simulink model "realtimeE4"  (R2024b)
settings: Solver=VariableStepAuto  StartTime=0.0  StopTime=10.0  RelTol=1e-3
values from neighbouring files (symbols this model uses):
  C = Tc/(Tc+Ts)    [Observer_and_complementary_filter.m]    (also in init.m = @(q) [)
undefined symbols (not defined in the file or in its folder): denH, denHw, DiscIntNeverNeededParam, drv, dspblkCoreblockFVToolHelper, gbox, gcbh, integral, numH, numHw, sens, Ts, wheel
settings Model: Creator=lucag  LastModifiedBy=lucag

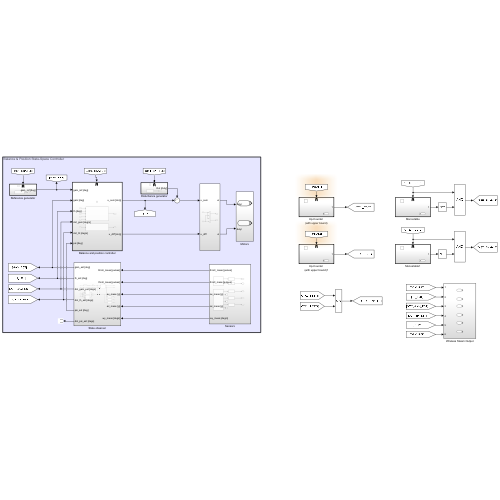
[thumbnail: Simulink's stored preview of the top-level diagram]
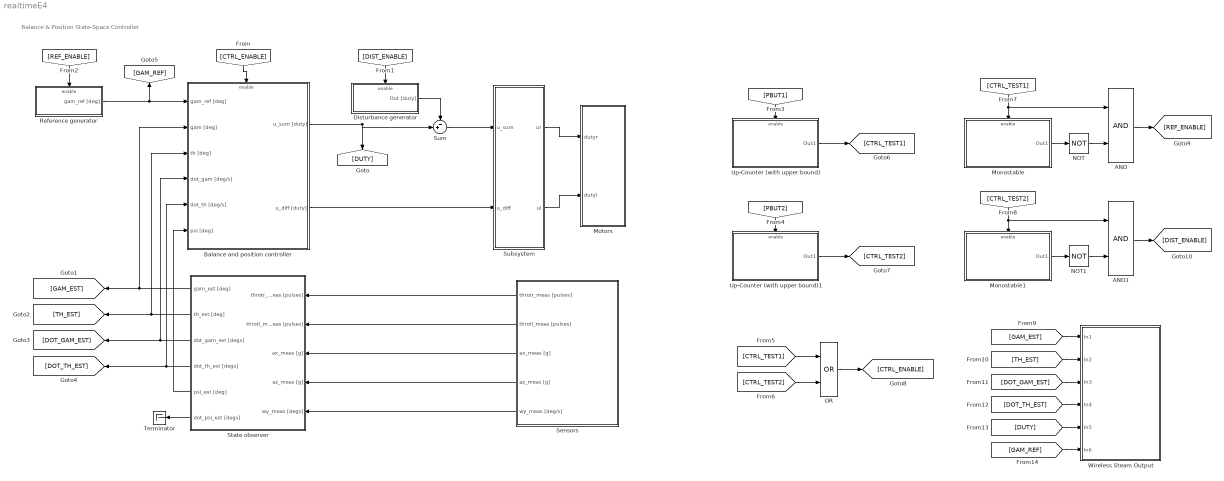
== system realtimeE4 ==
  note: Balance & Position State-Space Controller
  AND : Logic  AllPortsSameDT=off  OutDataTypeStr=boolean
  AND1 : Logic  AllPortsSameDT=off  OutDataTypeStr=boolean
  Balance and position controller : Subsystem  TreatAsAtomicUnit=on
  Disturbance generator : Subsystem  TreatAsAtomicUnit=on
  Monostable : Subsystem  TreatAsAtomicUnit=on
  Monostable1 : Subsystem  TreatAsAtomicUnit=on
  Motors : Subsystem
  NOT : Logic  Operator=NOT  AllPortsSameDT=off  OutDataTypeStr=boolean
  NOT1 : Logic  Operator=NOT  AllPortsSameDT=off  OutDataTypeStr=boolean
  OR : Logic  Operator=OR  AllPortsSameDT=off  OutDataTypeStr=boolean
  Reference generator : Subsystem  TreatAsAtomicUnit=on
  Sensors : Subsystem
  State observer : Subsystem
  Subsystem : Subsystem
  Sum : Sum  Inputs=-+|
  Terminator : Terminator
  Up-Counter (with upper bound) : Subsystem  TreatAsAtomicUnit=on
  Up-Counter (with upper bound)1 : Subsystem  TreatAsAtomicUnit=on
  Wireless Steam Output : Subsystem
  wires:
  [DUTY] -> Wireless Steam Output/5(In5)
  Up-Counter (with upper bound)/1(Out1) -> [CTRL_TEST1]
  [DOT_TH_EST] -> Wireless Steam Output/4(In4)
  AND1/1 -> [DIST_ENABLE]
  NOT/1 -> AND/2
  Monostable1/1(Out1) -> NOT1/1
  [PBUT2] -> Up-Counter (with upper bound)1/Enable
  AND/1 -> [REF_ENABLE]
  Up-Counter (with upper bound)1/1(Out1) -> [CTRL_TEST2]
  Sensors/1(throtr_meas [pulses]) -> State observer/1(throtr_meas [pulses])
  Sensors/5(wy_meas [deg/s]) -> State observer/5(wy_meas [degs])
  [DOT_GAM_EST] -> Wireless Steam Output/3(In3)
  Balance and position controller/1(u_sum [duty]) -> [DUTY], Sum/2
  Reference generator/1(gam_ref [deg]) -> Balance and position controller/1(gam_ref [deg]), [GAM_REF]
  [CTRL_TEST2] -> AND1/1, Monostable1/Enable
  [CTRL_ENABLE] -> Balance and position controller/Enable
  [CTRL_TEST2] -> OR/2
  [CTRL_TEST1] -> Monostable/Enable, AND/1
  State observer/1(gam_est [deg]) -> Balance and position controller/2(gam [deg]), [GAM_EST]
  Sensors/3(ax_meas [g]) -> State observer/3(ax_meas [g])
  NOT1/1 -> AND1/2
  [GAM_EST] -> Wireless Steam Output/1(In1)
  Disturbance generator/1(Out [duty]) -> Sum/1
  [DIST_ENABLE] -> Disturbance generator/Enable
  [PBUT1] -> Up-Counter (with upper bound)/Enable
  Monostable/1(Out1) -> NOT/1
  State observer/3(dot_gam_est [degs]) -> Balance and position controller/4(dot_gam [deg/s]), [DOT_GAM_EST]
  [REF_ENABLE] -> Reference generator/Enable
  OR/1 -> [CTRL_ENABLE]
  [CTRL_TEST1] -> OR/1
  State observer/4(dot_th_est [degs]) -> Balance and position controller/5(dot_th [deg/s]), [DOT_TH_EST]
  [GAM_REF] -> Wireless Steam Output/6(In6)
  Sensors/4(az_meas [g]) -> State observer/4(az_meas [g])
  [TH_EST] -> Wireless Steam Output/2(In2)
  State observer/2(th_est [deg]) -> Balance and position controller/3(th [deg]), [TH_EST]
  Sum/1 -> Subsystem/1(u_sum)
  Balance and position controller/2(u_diff [duty]) -> Subsystem/2(u_diff)
  Subsystem/1(ur) -> Motors/1(dutyr)
  Subsystem/2(ul) -> Motors/2(dutyl)
  Sensors/2(throtl_meas [pulses]) -> State observer/2(throtl_meas [pulses])
  State observer/5(psi_est [deg]) -> Balance and position controller/6(psi [deg])
  State observer/6(dot_psi_est [degs]) -> Terminator/1

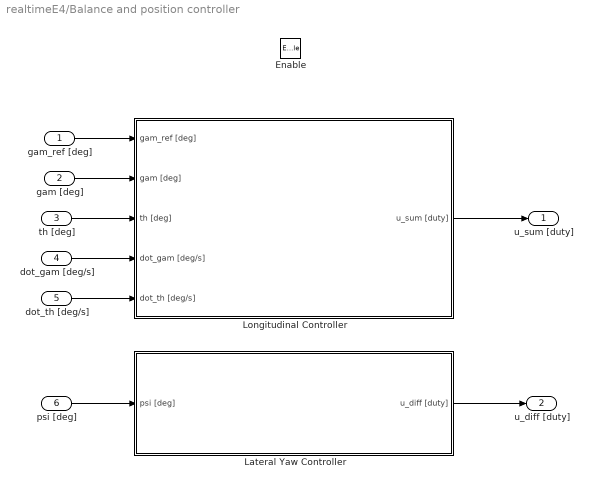
== system realtimeE4/Balance and position controller ==
  gam_ref [deg] : Inport
  gam [deg] : Inport  Port=2
  th [deg] : Inport  Port=3
  dot_gam [deg/s] : Inport  Port=4
  dot_th [deg/s] : Inport  Port=5
  psi [deg] : Inport  Port=6
  Enable : EnablePort
  Lateral Yaw Controller : Subsystem
  Longitudinal Controller : Subsystem
  u_sum [duty] : Outport  OutputWhenDisabled=reset
  u_diff [duty] : Outport  Port=2  OutputWhenDisabled=reset
  wires:
  dot_gam [deg/s]/1 -> Longitudinal Controller/4(dot_gam [deg/s])
  th [deg]/1 -> Longitudinal Controller/3(th [deg])
  gam [deg]/1 -> Longitudinal Controller/2(gam [deg])
  gam_ref [deg]/1 -> Longitudinal Controller/1(gam_ref [deg])
  Longitudinal Controller/1(u_sum [duty]) -> u_sum [duty]/1
  dot_th [deg/s]/1 -> Longitudinal Controller/5(dot_th [deg/s])
  psi [deg]/1 -> Lateral Yaw Controller/1(psi [deg])
  Lateral Yaw Controller/1(u_diff [duty]) -> u_diff [duty]/1

== system realtimeE4/Disturbance generator ==
  Enable : EnablePort
  Constant : Constant  Value=5.0/drv.duty2V
  Out [duty] : Outport  OutputWhenDisabled=reset
  wires:
  Constant/1 -> Out [duty]/1

== system realtimeE4/Monostable ==
  Enable : EnablePort
  Out1 : Outport

== system realtimeE4/Monostable1 ==
  Enable : EnablePort
  Out1 : Outport

== system realtimeE4/Motors ==
  dutyr : Inport
  dutyl : Inport  Port=2

== system realtimeE4/Reference generator ==
  Enable : EnablePort
  Constant : Constant  Value=(0.1/wheel.r)*rad2deg
  gam_ref [deg] : Outport  OutputWhenDisabled=reset
  wires:
  Constant/1 -> gam_ref [deg]/1

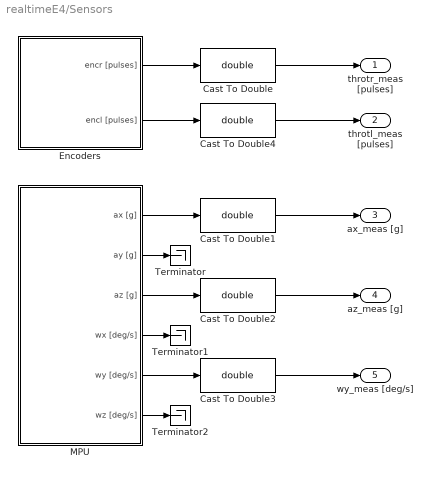
== system realtimeE4/Sensors ==
  Cast To Double{,1..4} (5 alike) : DataTypeConversion  OutDataTypeStr=double  SaturateOnIntegerOverflow=off  RndMeth=Floor
  Encoders : Subsystem
  MPU : Subsystem
  Terminator : Terminator
  Terminator1 : Terminator
  Terminator2 : Terminator
  throtr_meas [pulses] : Outport
  throtl_meas [pulses] : Outport  Port=2
  ax_meas [g] : Outport  Port=3
  az_meas [g] : Outport  Port=4
  wy_meas [deg/s] : Outport  Port=5
  wires:
  Cast To Double/1 -> throtr_meas [pulses]/1
  MPU/1(ax [g]) -> Cast To Double1/1
  MPU/3(az [g]) -> Cast To Double2/1
  MPU/5(wy [deg/s]) -> Cast To Double3/1
  MPU/2(ay [g]) -> Terminator/1
  MPU/4(wx [deg/s]) -> Terminator1/1
  MPU/6(wz [deg/s]) -> Terminator2/1
  Cast To Double1/1 -> ax_meas [g]/1
  Cast To Double2/1 -> az_meas [g]/1
  Cast To Double3/1 -> wy_meas [deg/s]/1
  Encoders/1(encr [pulses]) -> Cast To Double/1
  Encoders/2(encl [pulses]) -> Cast To Double4/1
  Cast To Double4/1 -> throtl_meas [pulses]/1

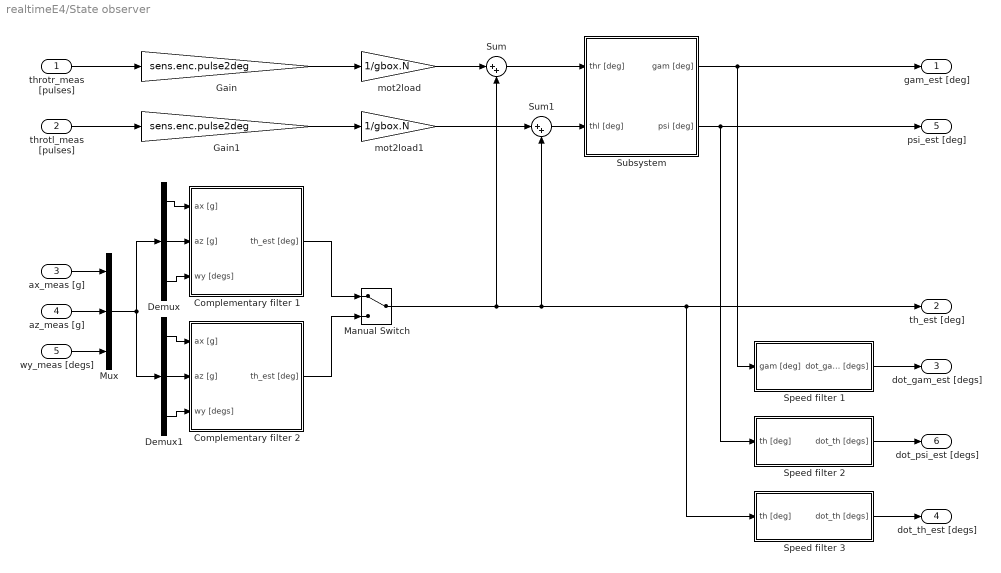
== system realtimeE4/State observer ==
  throtr_meas [pulses] : Inport
  throtl_meas [pulses] : Inport  Port=2
  ax_meas [g] : Inport  Port=3
  az_meas [g] : Inport  Port=4
  wy_meas [degs] : Inport  Port=5
  Complementary filter 1 : Subsystem
  Complementary filter 2 : Subsystem
  Demux : Demux  Outputs=3
  Demux1 : Demux  Outputs=3
  Gain : Gain  Gain=sens.enc.pulse2deg
  Gain1 : Gain  Gain=sens.enc.pulse2deg
  Manual Switch : ManualSwitch
  Mux : Mux  Inputs=3
  Speed filter 1 : Subsystem
  Speed filter 2 : Subsystem
  Speed filter 3 : Subsystem
  Subsystem : Subsystem
  Sum : Sum  Inputs=|++
  Sum1 : Sum  Inputs=|++
  mot2load : Gain  Gain=1/gbox.N
  mot2load1 : Gain  Gain=1/gbox.N
  gam_est [deg] : Outport
  th_est [deg] : Outport  Port=2
  dot_gam_est [degs] : Outport  Port=3
  dot_th_est [degs] : Outport  Port=4
  psi_est [deg] : Outport  Port=5
  dot_psi_est [degs] : Outport  Port=6
  wires:
  throtr_meas [pulses]/1 -> Gain/1
  Gain/1 -> mot2load/1
  mot2load/1 -> Sum/1
  Speed filter 1/1(dot_gam [degs]) -> dot_gam_est [degs]/1
  ax_meas [g]/1 -> Mux/1
  az_meas [g]/1 -> Mux/2
  wy_meas [degs]/1 -> Mux/3
  Demux/1 -> Complementary filter 1/1(ax [g])
  Demux/3 -> Complementary filter 1/3(wy [degs])
  Demux/2 -> Complementary filter 1/2(az [g])
  Demux1/2 -> Complementary filter 2/2(az [g])
  Demux1/1 -> Complementary filter 2/1(ax [g])
  Demux1/3 -> Complementary filter 2/3(wy [degs])
  Mux/1 -> Demux/1, Demux1/1
  Complementary filter 1/1(th_est [deg]) -> Manual Switch/1
  Complementary filter 2/1(th_est [deg]) -> Manual Switch/2
  Manual Switch/1 -> Sum/2, Sum1/2, Speed filter 3/1(th [deg]), th_est [deg]/1
  throtl_meas [pulses]/1 -> Gain1/1
  Gain1/1 -> mot2load1/1
  mot2load1/1 -> Sum1/1
  Sum/1 -> Subsystem/1(thr [deg])
  Sum1/1 -> Subsystem/2(thl [deg])
  Subsystem/1(gam [deg]) -> Speed filter 1/1(gam [deg]), gam_est [deg]/1
  Subsystem/2(psi [deg]) -> Speed filter 2/1(th [deg]), psi_est [deg]/1
  Speed filter 3/1(dot_th [degs]) -> dot_th_est [degs]/1
  Speed filter 2/1(dot_th [degs]) -> dot_psi_est [degs]/1

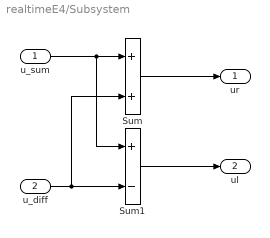
== system realtimeE4/Subsystem ==
  u_sum : Inport
  u_diff : Inport  Port=2
  Sum : Sum
  Sum1 : Sum  Inputs=+-
  ur : Outport
  ul : Outport  Port=2
  wires:
  u_sum/1 -> Sum1/1, Sum/1
  u_diff/1 -> Sum/2, Sum1/2
  Sum/1 -> ur/1
  Sum1/1 -> ul/1

== system realtimeE4/Up-Counter (with upper bound) ==
  Enable : EnablePort
  Out1 : Outport

== system realtimeE4/Up-Counter (with upper bound)1 ==
  Enable : EnablePort
  Out1 : Outport

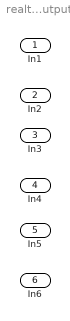
== system realtimeE4/Wireless Steam Output ==
  In1 : Inport
  In2 : Inport  Port=2
  In3 : Inport  Port=3
  In4 : Inport  Port=4
  In5 : Inport  Port=5
  In6 : Inport  Port=6

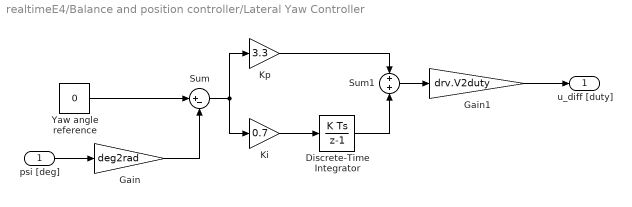
== system realtimeE4/Balance and position controller/Lateral Yaw Controller ==
  psi [deg] : Inport
  Discrete-Time Integrator : DiscreteIntegrator  SampleTime=-1  ICPrevOutput=DiscIntNeverNeededParam  ICPrevScaledInput=DiscIntNeverNeededParam
  Gain : Gain  Gain=deg2rad
  Gain1 : Gain  Gain=drv.V2duty
  Ki : Gain  Gain=0.7
  Kp : Gain  Gain=3.3
  Sum : Sum  Inputs=|+-
  Sum1 : Sum
  Yaw angle reference : Constant  Value=0
  u_diff [duty] : Outport
  wires:
  psi [deg]/1 -> Gain/1
  Yaw angle reference/1 -> Sum/1
  Gain/1 -> Sum/2
  Sum/1 -> Kp/1, Ki/1
  Ki/1 -> Discrete-Time Integrator/1
  Kp/1 -> Sum1/1
  Discrete-Time Integrator/1 -> Sum1/2
  Sum1/1 -> Gain1/1
  Gain1/1 -> u_diff [duty]/1

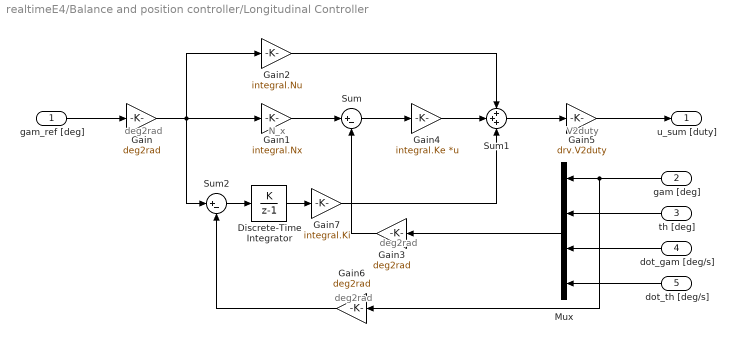
== system realtimeE4/Balance and position controller/Longitudinal Controller ==
  note: deg2rad
  note: N_x
  note: V2duty
  note: deg2rad
  note: deg2rad
  gam_ref [deg] : Inport
  gam [deg] : Inport  Port=2
  th [deg] : Inport  Port=3
  dot_gam [deg/s] : Inport  Port=4
  dot_th [deg/s] : Inport  Port=5
  Discrete-Time Integrator : DiscreteIntegrator  IntegratorMethod=Accumulation: Forward Euler  SampleTime=Ts  ICPrevOutput=DiscIntNeverNeededParam  ICPrevScaledInput=DiscIntNeverNeededParam
  Gain : Gain  Gain=deg2rad
  Gain1 : Gain  Gain=integral.Nx
  Gain2 : Gain  Gain=integral.Nu
  Gain3 : Gain  Gain=deg2rad
  Gain4 : Gain  Gain=integral.Ke  Multiplication=Matrix(K*u)
  Gain5 : Gain  Gain=drv.V2duty
  Gain6 : Gain  Gain=deg2rad
  Gain7 : Gain  Gain=integral.Ki
  Mux : Mux
  Sum : Sum  Inputs=|+-
  Sum1 : Sum  Inputs=+++
  Sum2 : Sum  Inputs=|+-
  u_sum [duty] : Outport
  wires:
  Discrete-Time Integrator/1 -> Gain7/1
  gam [deg]/1 -> Gain6/1, Mux/1
  Mux/1 -> Gain3/1
  Gain6/1 -> Sum2/2
  Gain/1 -> Sum2/1, Gain2/1, Gain1/1
  gam_ref [deg]/1 -> Gain/1
  dot_gam [deg/s]/1 -> Mux/3
  Sum/1 -> Gain4/1
  Gain7/1 -> Sum1/3
  Sum1/1 -> Gain5/1
  Gain1/1 -> Sum/1
  Gain2/1 -> Sum1/1
  Gain4/1 -> Sum1/2
  Gain3/1 -> Sum/2
  Sum2/1 -> Discrete-Time Integrator/1
  th [deg]/1 -> Mux/2
  dot_th [deg/s]/1 -> Mux/4
  Gain5/1 -> u_sum [duty]/1

== system realtimeE4/Sensors/Encoders ==
  encr [pulses] : Outport
  encl [pulses] : Outport  Port=2

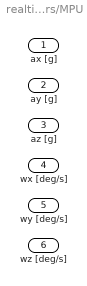
== system realtimeE4/Sensors/MPU ==
  ax [g] : Outport
  ay [g] : Outport  Port=2
  az [g] : Outport  Port=3
  wx [deg/s] : Outport  Port=4
  wy [deg/s] : Outport  Port=5
  wz [deg/s] : Outport  Port=6

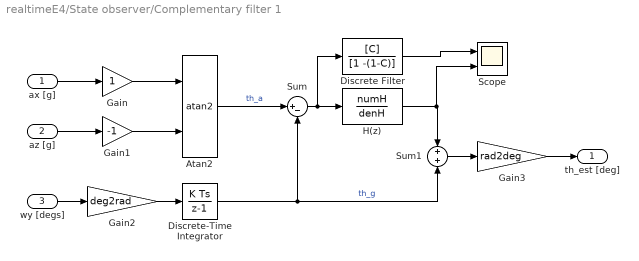
== system realtimeE4/State observer/Complementary filter 1 ==
  ax [g] : Inport
  az [g] : Inport  Port=2
  wy [degs] : Inport  Port=3
  Atan2 : Trigonometry  Operator=atan2
  Discrete Filter : DiscreteFilter  LoadFcn=dspblkCoreblockFVToolHelper(gcbh,'load');  Numerator=[C]  Denominator=[1 -(1-C)]
      settings: CopyFcn=dspblkCoreblockFVToolHelper(gcbh,'copy');  DeleteFcn=dspblkCoreblockFVToolHelper(gcbh,'close');  ModelCloseFcn=dspblkCoreblockFVToolHelper(gcbh,'close');  PreSaveFcn=dspblkCoreblockFVToolHelper(gcbh,'presave');  PostSaveFcn=dspblkCoreblockFVToolHelper(gcbh,'postsave');  CloseFcn=dspblkCoreblockFVToolHelper(gcbh,'close');
  Discrete-Time Integrator : DiscreteIntegrator  SampleTime=Ts  ICPrevOutput=DiscIntNeverNeededParam  ICPrevScaledInput=DiscIntNeverNeededParam
  Gain : Gain
  Gain1 : Gain  Gain=-1
  Gain2 : Gain  Gain=deg2rad
  Gain3 : Gain  Gain=rad2deg
  H(z) : DiscreteTransferFcn  Numerator=numH  Denominator=denH
  Scope : Scope  NumInputPorts=2
  Sum : Sum  Inputs=|+-
  Sum1 : Sum  Inputs=+|+
  th_est [deg] : Outport
  wires:
  ax [g]/1 -> Gain/1
  az [g]/1 -> Gain1/1
  Gain/1 -> Atan2/1
  Gain1/1 -> Atan2/2
  Atan2/1 -> Sum/1  "th_a"
  wy [degs]/1 -> Gain2/1
  Gain2/1 -> Discrete-Time Integrator/1
  Discrete-Time Integrator/1 -> Sum1/2, Sum/2  "th_g"
  Sum/1 -> Discrete Filter/1, H(z)/1
  H(z)/1 -> Scope/2, Sum1/1
  Sum1/1 -> Gain3/1
  Gain3/1 -> th_est [deg]/1
  Discrete Filter/1 -> Scope/1

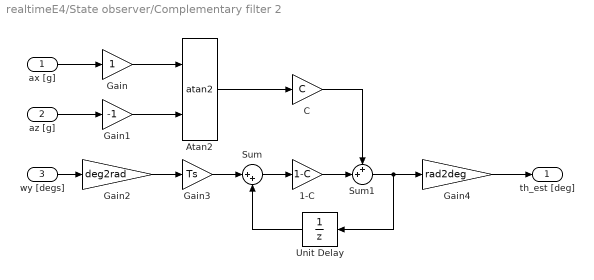
== system realtimeE4/State observer/Complementary filter 2 ==
  ax [g] : Inport
  az [g] : Inport  Port=2
  wy [degs] : Inport  Port=3
  1-C : Gain  Gain=1-C
  Atan2 : Trigonometry  Operator=atan2
  C : Gain  Gain=C
  Gain : Gain
  Gain1 : Gain  Gain=-1
  Gain2 : Gain  Gain=deg2rad
  Gain3 : Gain  Gain=Ts
  Gain4 : Gain  Gain=rad2deg
  Sum : Sum  Inputs=|++
  Sum1 : Sum  Inputs=++|
  Unit Delay : UnitDelay  SampleTime=-1  HasFrameUpgradeWarning=on
  th_est [deg] : Outport
  wires:
  Gain/1 -> Atan2/1
  az [g]/1 -> Gain1/1
  Gain1/1 -> Atan2/2
  ax [g]/1 -> Gain/1
  Atan2/1 -> C/1
  wy [degs]/1 -> Gain2/1
  Gain2/1 -> Gain3/1
  Gain3/1 -> Sum/1
  Sum/1 -> 1-C/1
  C/1 -> Sum1/1
  1-C/1 -> Sum1/2
  Sum1/1 -> Unit Delay/1, Gain4/1
  Unit Delay/1 -> Sum/2
  Gain4/1 -> th_est [deg]/1

== system realtimeE4/State observer/Speed filter 1 ==
  gam [deg] : Inport
  Discrete Transfer Fcn : DiscreteTransferFcn  Numerator=numHw  Denominator=denHw
  Discrete Filter : DiscreteFilter  LoadFcn=dspblkCoreblockFVToolHelper(gcbh,'load');  Numerator=[1 0 0 -1]  Denominator=[3*Ts,0,0,0]  SampleTime=Ts
      settings: CopyFcn=dspblkCoreblockFVToolHelper(gcbh,'copy');  DeleteFcn=dspblkCoreblockFVToolHelper(gcbh,'close');  ModelCloseFcn=dspblkCoreblockFVToolHelper(gcbh,'close');  PreSaveFcn=dspblkCoreblockFVToolHelper(gcbh,'presave');  PostSaveFcn=dspblkCoreblockFVToolHelper(gcbh,'postsave');  CloseFcn=dspblkCoreblockFVToolHelper(gcbh,'close');
  Scope : Scope  NumInputPorts=2
  dot_gam [degs] : Outport
  wires:
  gam [deg]/1 -> Discrete Filter/1, Discrete Transfer Fcn/1
  Discrete Transfer Fcn/1 -> Scope/1, dot_gam [degs]/1
  Discrete Filter/1 -> Scope/2

== system realtimeE4/State observer/Speed filter 2 ==
  th [deg] : Inport
  Discrete Transfer Fcn : DiscreteTransferFcn  Numerator=numHw  Denominator=denHw
  dot_th [degs] : Outport
  wires:
  th [deg]/1 -> Discrete Transfer Fcn/1
  Discrete Transfer Fcn/1 -> dot_th [degs]/1

== system realtimeE4/State observer/Speed filter 3 ==
  th [deg] : Inport
  Discrete Transfer Fcn : DiscreteTransferFcn  Numerator=numHw  Denominator=denHw
  dot_th [degs] : Outport
  wires:
  Discrete Transfer Fcn/1 -> dot_th [degs]/1
  th [deg]/1 -> Discrete Transfer Fcn/1

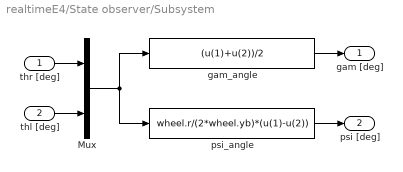
== system realtimeE4/State observer/Subsystem ==
  thr [deg] : Inport
  thl [deg] : Inport  Port=2
  Mux : Mux  Inputs=2
  gam_angle : Fcn  Expr=(u(1)+u(2))/2
  psi_angle : Fcn  Expr=wheel.r/(2*wheel.yb)*(u(1)-u(2))
  gam [deg] : Outport
  psi [deg] : Outport  Port=2
  wires:
  thr [deg]/1 -> Mux/1
  thl [deg]/1 -> Mux/2
  Mux/1 -> psi_angle/1, gam_angle/1
  gam_angle/1 -> gam [deg]/1
  psi_angle/1 -> psi [deg]/1
